simulink model "Position_augment_Testing"  (R2018a)
settings: Solver=VariableStepAuto  StartTime=0.0  StopTime=inf  RelTol=1e-3
undefined symbols (not defined in the file): Ad, Bd, Beta, C1, C2, cBW, d, dw, I, Iw, Kb, Kg, Kt, La, mc, R, Ra, sampleTime, Waypoint
libraries: cstblocks x3, mobileRoboticsLib x2, dspsrcs4 x1
settings Model: Creator=shravan  LastModifiedBy=shravan

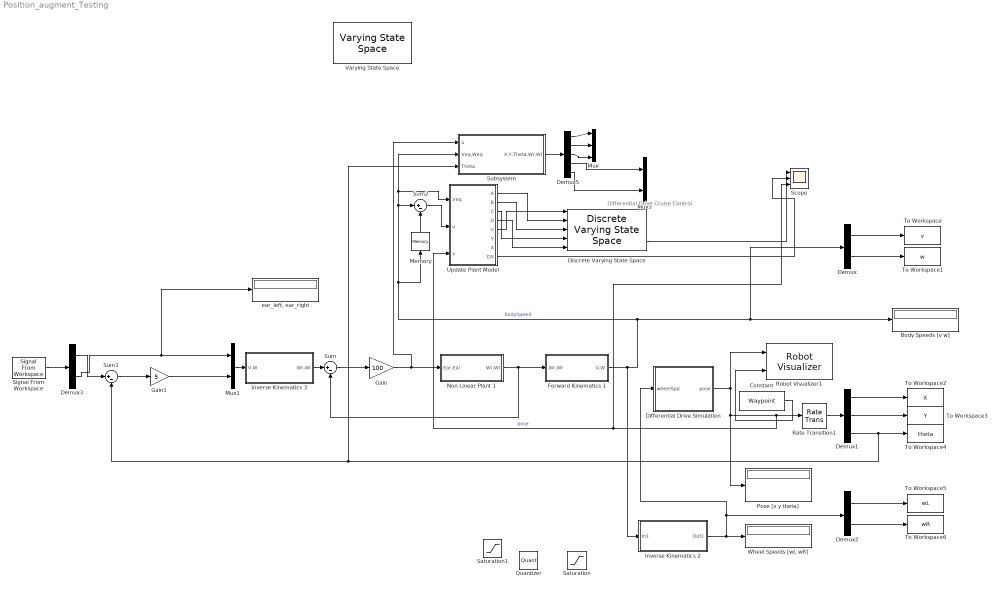
== system Position_augment_Testing ==
  note: Differential Drive Cruise Control
  Body Speeds [v w] : Display
  Constant : Constant  Value=Waypoint  SampleTime=sampleTime
  Demux : Demux  Outputs=2
  Demux1 : Demux  Outputs=3
  Demux2 : Demux  Outputs=2
  Demux3 : Demux  Outputs=2
  Demux5 : Demux  Outputs=5
  Differential Drive Simulation : Subsystem  AncestorBlock=mobileRoboticsLib/Kinematic Models/Differential Drive/Differential Drive Simulation  OverrideUsingVariant=mode==2  mask(Differential Drive Simulation){wheelRadius=R, wheelBase=dw, initX=C1, initY=C2, initAngle=0, Ts=sampleTime}
      mask prompts: wheelRadius "Wheel Radius [m]"; wheelBase "Wheelbase [m]"; initX "Initial X Position [m]"; initY "Initial Y Position [m]"; initAngle "Initial Angle [rad]"; Ts "Sample Time"
      mask help:
      | Simulates the kinematics of a differential drive vehicle from a specified initial pose.
      |
      | Input: Left and right wheel speeds [wL; wR], in rad/s
      |
      | Output: Pose [x; y; theta], in m, m, and rad
      |
      | Set the Sample Time parameter to 0 for continuous-time simulation, or a positive number for discrete-time simulation.
      mask Help: web('matlab:edit mrsDocDifferentialDrive')
      mask Callback Ts:
      | Ts = evalin('base',get_param(gcb,'Ts'));
      | blk = [gcb '/Generic Robot Simulation/Velocity Integrator'];
      | if Ts > 0
      |     set_param(blk,'OverrideUsingVariant','mode==2');
      | else
      |     set_param(blk,'OverrideUsingVariant','mode==1');
      | end
  Discrete Varying State Space : cstblocks/Linear Parameter Varying/Discrete Varying State Space  x0=[C1 C2 0]'  Ts=-1  OutputX=on  OutputDX=on
      settings: SourceProductName=Control System Toolbox  SourceProductBaseCode=CT
  Forward Kinematics 1 : Subsystem
  Gain : Gain  Gain=100
  Gain1 : Gain  Gain=5
  Inverse Kinematics 2 : Subsystem
  Inverse Kinematics 3 : Subsystem
  Memory : Memory
  Mux : Mux  Inputs=3
  Mux1 : Mux  Inputs=2
  Mux3 : Mux  Inputs=2
  Non Linear Plant 1 : Subsystem
  Pose [x y theta] : Display
  Quantizer : Quantizer
  Rate Transition1 : RateTransition  OutPortSampleTime=sampleTime
  Robot Visualizer1 : mobileRoboticsLib/Environments/Robot Visualizer  Priority=99  robotRadius=1  showTrajectory=on  hasWaypoints=on  hasLidar=off  sensorOffset=[ 0 0 ]  scanAngles=[-pi/4,0,pi/4]  hasObjDetector=off  objDetectorOffset=[ 0, 0 ]  objDetectorAngle=0  objDetectorFOV=pi/4  objDetectorMaxRange=5  objectColors=[ 1, 0, 0; 0, 1, 0; 0, 0, 1 ]  objectMarkers='s'
      settings: SourceProductName=Mobile Robotics Simulation Library
  Saturation : Saturate
  Saturation1 : Saturate  UpperLimit=12  LowerLimit=0
  Scope : Scope  NumInputPorts=3
  Signal From Workspace : dspsrcs4/Signal From Workspace  X=Cruise  Ts=cBW  nsamps=1  OutputAfterFinalValue=Holding final value  ignoreOrWarnInputAndFrameLengths=off  OutputFrames=off
  Subsystem : Subsystem
  Sum : Sum  Inputs=|+-
  Sum1 : Sum  Inputs=|+-
  Sum2 : Sum  Inputs=|+-
  To Workspace : ToWorkspace  VariableName=v  SampleTime=-1
  To Workspace1 : ToWorkspace  VariableName=w  SampleTime=-1
  To Workspace2 : ToWorkspace  VariableName=X  SampleTime=-1
  To Workspace3 : ToWorkspace  VariableName=Y  SampleTime=-1
  To Workspace4 : ToWorkspace  VariableName=theta  SampleTime=-1
  To Workspace5 : ToWorkspace  VariableName=wL  SampleTime=-1
  To Workspace6 : ToWorkspace  VariableName=wR  SampleTime=-1
  Update Plant Model : MATLAB Function  TreatAsAtomicUnit=on  SystemSampleTime=0
  Varying State Space : cstblocks/Linear Parameter Varying/Varying State Space  x0=0  xNames=''  OutputX=on  OutputDX=on
      settings: SourceProductName=Control System Toolbox
  Wheel Speeds [wL wR] : Display
  "ear_left, ear_right " : Display
  wires:
  Constant/1 -> Robot Visualizer1/2
  Differential Drive Simulation/1(pose) -> Robot Visualizer1/1, Scope/3, Update Plant Model/3(x), Rate Transition1/1, Pose [x y theta]/1  "pose"
  Sum1/1 -> Gain1/1
  Demux/1 -> To Workspace/1
  Demux/2 -> To Workspace1/1
  Demux2/1 -> To Workspace5/1
  Inverse Kinematics 3/1(Wr,Wl) -> Sum/1
  Demux1/2 -> To Workspace3/1
  Demux3/2 -> "ear_left, ear_right "/1, Mux1/1
  Rate Transition1/1 -> Demux1/1
  Forward Kinematics 1/1(V,W) -> Inverse Kinematics 2/1(In1), Memory/1, Sum2/1, Update Plant Model/1(Veq), Subsystem/2("Veq,Weq "), Demux/1, Body Speeds [v w]/1  "bodySpeed"
  Gain1/1 -> Mux1/2
  Demux2/2 -> To Workspace6/1
  Demux3/1 -> Sum1/1
  Mux1/1 -> Inverse Kinematics 3/1(V,W)
  Inverse Kinematics 2/1(Out1) -> Differential Drive Simulation/1(wheelSpd), Demux2/1, Wheel Speeds [wL wR]/1
  Demux1/1 -> To Workspace2/1
  Signal From Workspace/1 -> Demux3/1
  Subsystem/1(X,Y,Theta,Wr,Wl) -> Demux5/1
  Demux5/2 -> Mux/2
  Demux5/1 -> Mux/1
  Demux5/3 -> Mux/3
  Sum/1 -> Gain/1
  Demux5/5 -> Mux3/2
  Demux5/4 -> Mux3/1
  Gain/1 -> Subsystem/1("u "), Non Linear Plant 1/1("Ear,Eal ")
  Demux1/3 -> Subsystem/3("Theta "), Sum1/2, To Workspace4/1
  Non Linear Plant 1/1(Wr,Wl) -> Sum/2, Forward Kinematics 1/1(Wr,Wl)
  Update Plant Model/1(A) -> Discrete Varying State Space/2
  Update Plant Model/2(B) -> Discrete Varying State Space/3
  Update Plant Model/3(C) -> Discrete Varying State Space/4
  Update Plant Model/4(D) -> Discrete Varying State Space/5
  Update Plant Model/5(U) -> Discrete Varying State Space/1
  Memory/1 -> Sum2/2
  Sum2/1 -> Update Plant Model/2(u)
  Discrete Varying State Space/3 -> Scope/1
  Update Plant Model/8(DX) -> Scope/2

== system Position_augment_Testing/Differential Drive Simulation ==
  wheelSpd : Inport
  Constant : Constant  Value=0
  Demux : Demux  Outputs=2
  "Forward Kinematics " : Subsystem
  Generic Robot Simulation : mobileRoboticsLib/Utilities/Generic Vehicle Simulation  initX=initX  initY=initY  initAngle=initAngle  Ts=Ts
      link override Velocity Integrator: OverrideUsingVariant=mode==2
      settings: SourceProductName=Mobile Robotics Simulation Toolbox
  Mux1 : Mux  Inputs=3
  pose : Outport
  wires:
  Generic Robot Simulation/1 -> pose/1
  "Forward Kinematics "/1(Out1) -> Demux/1
  wheelSpd/1 -> "Forward Kinematics "/1(In1)
  Constant/1 -> Mux1/2  "vy"
  Demux/2 -> Mux1/3  "w"
  Demux/1 -> Mux1/1  "vx"
  Mux1/1 -> Generic Robot Simulation/1

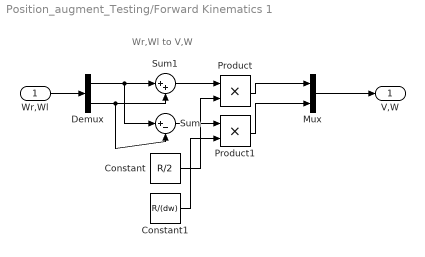
== system Position_augment_Testing/Forward Kinematics 1 ==
  note: Wr,Wl to V,W
  Wr,Wl : Inport
  Constant : Constant  Value=R/2
  Constant1 : Constant  Value=R/(dw)
  Demux : Demux  Outputs=2
  Mux : Mux  Inputs=2
  Product : Product
  Product1 : Product
  Sum : Sum  Inputs=|+-
  Sum1 : Sum  Inputs=|++
  V,W : Outport
  wires:
  Constant1/1 -> Product1/2
  Sum/1 -> Product1/1
  Constant/1 -> Product/2
  Sum1/1 -> Product/1
  Demux/2 -> Sum1/2, Sum/2
  Demux/1 -> Sum1/1, Sum/1
  Product/1 -> Mux/1
  Mux/1 -> V,W/1
  Product1/1 -> Mux/2
  Wr,Wl/1 -> Demux/1

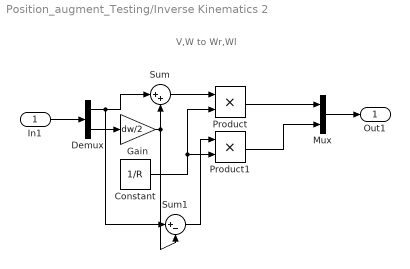
== system Position_augment_Testing/Inverse Kinematics 2 ==
  note: V,W to Wr,Wl
  In1 : Inport
  Constant : Constant  Value=1/R
  Demux : Demux  Outputs=2
  Gain : Gain  Gain=dw/2
  Mux : Mux  Inputs=2
  Product : Product
  Product1 : Product
  Sum : Sum  Inputs=|++
  Sum1 : Sum  Inputs=|+-
  Out1 : Outport
  wires:
  Gain/1 -> Sum/2, Sum1/2
  Product1/1 -> Mux/2
  Product/1 -> Mux/1
  Sum1/1 -> Product1/1
  Constant/1 -> Product/2, Product1/2
  Sum/1 -> Product/1
  Demux/1 -> Sum/1, Sum1/1
  Demux/2 -> Gain/1
  In1/1 -> Demux/1
  Mux/1 -> Out1/1

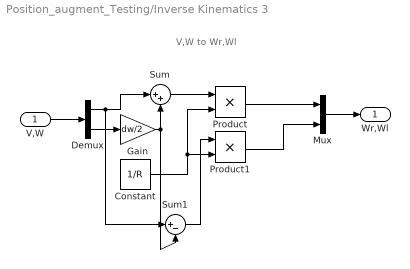
== system Position_augment_Testing/Inverse Kinematics 3 ==
  note: V,W to Wr,Wl
  V,W : Inport
  Constant : Constant  Value=1/R
  Demux : Demux  Outputs=2
  Gain : Gain  Gain=dw/2
  Mux : Mux  Inputs=2
  Product : Product
  Product1 : Product
  Sum : Sum  Inputs=|++
  Sum1 : Sum  Inputs=|+-
  Wr,Wl : Outport
  wires:
  Gain/1 -> Sum/2, Sum1/2
  Product1/1 -> Mux/2
  Product/1 -> Mux/1
  Sum1/1 -> Product1/1
  Constant/1 -> Product/2, Product1/2
  Sum/1 -> Product/1
  Demux/1 -> Sum/1, Sum1/1
  Demux/2 -> Gain/1
  V,W/1 -> Demux/1
  Mux/1 -> Wr,Wl/1

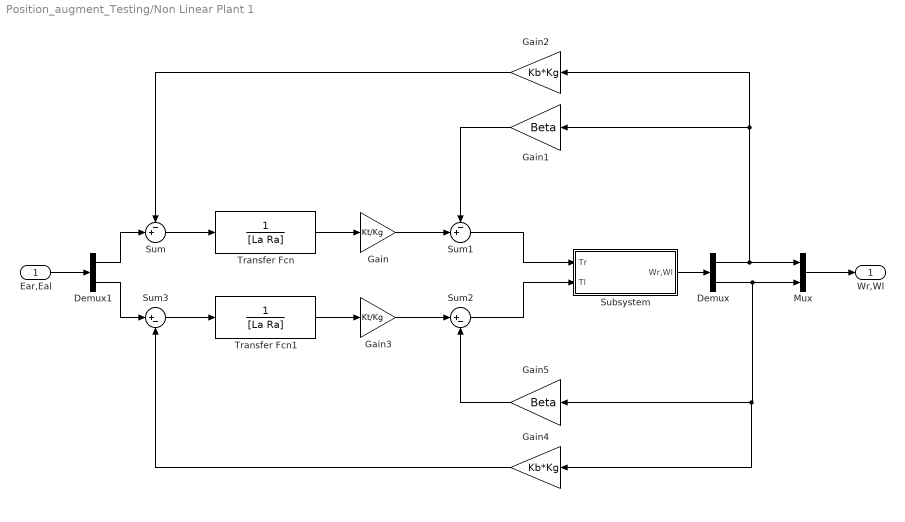
== system Position_augment_Testing/Non Linear Plant 1 ==
  "Ear,Eal " : Inport
  Demux : Demux  Outputs=2
  Demux1 : Demux  Outputs=2
  Gain : Gain  Gain=Kt/Kg
  Gain1 : Gain  Gain=Beta
  Gain2 : Gain  Gain=Kb*Kg
  Gain3 : Gain  Gain=Kt/Kg
  Gain4 : Gain  Gain=Kb*Kg
  Gain5 : Gain  Gain=Beta
  Mux : Mux  Inputs=2
  Subsystem : Subsystem
  Sum : Sum  Inputs=-+|
  Sum1 : Sum  Inputs=-+|
  Sum2 : Sum  Inputs=|+-
  Sum3 : Sum  Inputs=|+-
  Transfer Fcn : TransferFcn  Denominator=[La Ra]
  Transfer Fcn1 : TransferFcn  Denominator=[La Ra]
  Wr,Wl : Outport
  wires:
  Sum2/1 -> Subsystem/2(Tl)
  Demux/2 -> Gain5/1, Gain4/1, Mux/2
  Gain3/1 -> Sum2/1
  Transfer Fcn1/1 -> Gain3/1
  Transfer Fcn/1 -> Gain/1
  Sum1/1 -> Subsystem/1(Tr)
  "Ear,Eal "/1 -> Demux1/1
  Gain/1 -> Sum1/2
  Gain2/1 -> Sum/1
  Mux/1 -> Wr,Wl/1
  Sum3/1 -> Transfer Fcn1/1
  Demux1/1 -> Sum/2
  Subsystem/1(Wr,Wl) -> Demux/1
  Demux/1 -> Gain1/1, Gain2/1, Mux/1
  Gain1/1 -> Sum1/1
  Demux1/2 -> Sum3/1
  Sum/1 -> Transfer Fcn/1
  Gain4/1 -> Sum3/2
  Gain5/1 -> Sum2/2

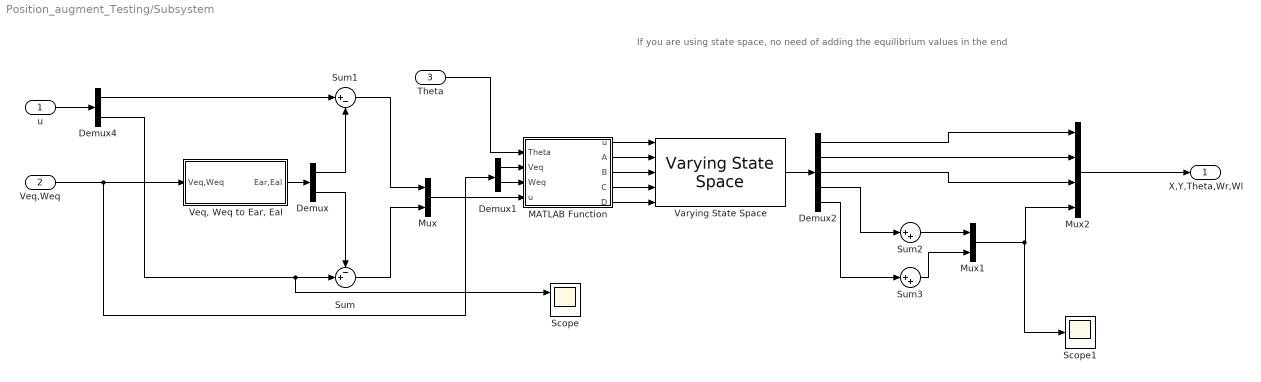
== system Position_augment_Testing/Subsystem ==
  note: If you are using state space, no need of adding the equilibrium values in the end
  "u " : Inport
  "Veq,Weq " : Inport  Port=2
  "Theta " : Inport  Port=3
  Demux : Demux  Outputs=2
  Demux1 : Demux  Outputs=2
  Demux2 : Demux  Outputs=5
  Demux4 : Demux  Outputs=2
  MATLAB Function : MATLAB Function  TreatAsAtomicUnit=on  SystemSampleTime=sampleTime*0.1
  Mux : Mux  Inputs=2
  Mux1 : Mux  Inputs=2
  Mux2 : Mux
  Scope : Scope  NumInputPorts=2
  Scope1 : Scope
  Sum : Sum  Inputs=-+|
  Sum1 : Sum  Inputs=|+-
  Sum2 : Sum  Inputs=|++
  Sum3 : Sum  Inputs=|++
  Varying State Space : cstblocks/Linear Parameter Varying/Varying State Space  x0=[C1;C2;0;0;0;0;0]  xNames=''  OutputX=off  OutputDX=off
      settings: SourceProductName=Control System Toolbox
  "Veq, Weq to Ear, Eal " : Subsystem
  X,Y,Theta,Wr,Wl : Outport
  wires:
  "Veq, Weq to Ear, Eal "/1(Ear,Eal) -> Demux/1
  Demux/1 -> Sum1/2
  Demux/2 -> Sum/1
  MATLAB Function/3(B) -> Varying State Space/3
  MATLAB Function/4(C) -> Varying State Space/4
  MATLAB Function/1(u) -> Varying State Space/1
  MATLAB Function/2(A) -> Varying State Space/2
  MATLAB Function/5(D) -> Varying State Space/5
  Sum1/1 -> Mux/1
  Sum/1 -> Mux/2
  Mux/1 -> MATLAB Function/4("u ")
  "Theta "/1 -> MATLAB Function/1(Theta)
  Demux1/2 -> MATLAB Function/3(Weq)
  Demux1/1 -> MATLAB Function/2(Veq)
  Varying State Space/1 -> Demux2/1
  Demux2/1 -> Mux2/1
  Demux2/2 -> Mux2/2
  Demux2/3 -> Mux2/3
  Demux2/4 -> Sum2/1
  Demux2/5 -> Sum3/1
  Mux1/1 -> Scope1/1, Mux2/4
  Sum2/1 -> Mux1/1
  Sum3/1 -> Mux1/2
  "Veq,Weq "/1 -> "Veq, Weq to Ear, Eal "/1(Veq,Weq), Demux1/1
  Mux2/1 -> X,Y,Theta,Wr,Wl/1
  "u "/1 -> Demux4/1
  Demux4/1 -> Sum1/1
  Demux4/2 -> Scope/1, Sum/2

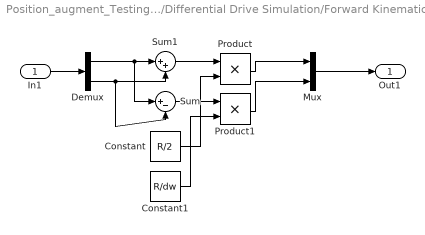
== system Position_augment_Testing/Differential Drive Simulation/Forward Kinematics  ==
  In1 : Inport
  Constant : Constant  Value=R/2
  Constant1 : Constant  Value=R/dw
  Demux : Demux  Outputs=2
  Mux : Mux  Inputs=2
  Product : Product
  Product1 : Product
  Sum : Sum  Inputs=|+-
  Sum1 : Sum  Inputs=|++
  Out1 : Outport
  wires:
  In1/1 -> Demux/1
  Product1/1 -> Mux/2
  Mux/1 -> Out1/1
  Product/1 -> Mux/1
  Demux/1 -> Sum/1, Sum1/1
  Demux/2 -> Sum/2, Sum1/2
  Sum1/1 -> Product/1
  Constant/1 -> Product/2
  Sum/1 -> Product1/1
  Constant1/1 -> Product1/2

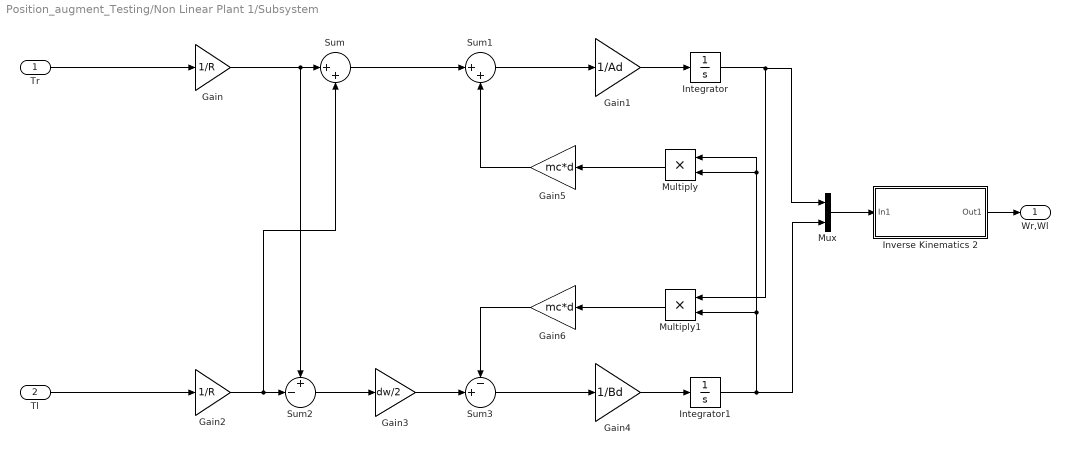
== system Position_augment_Testing/Non Linear Plant 1/Subsystem ==
  Tr : Inport
  Tl : Inport  Port=2
  Gain : Gain  Gain=1/R
  Gain1 : Gain  Gain=1/Ad
  Gain2 : Gain  Gain=1/R
  Gain3 : Gain  Gain=dw/2
  Gain4 : Gain  Gain=1/Bd
  Gain5 : Gain  Gain=mc*d
  Gain6 : Gain  Gain=mc*d
  Integrator : Integrator
  Integrator1 : Integrator
  Inverse Kinematics 2 : Subsystem
  Multiply : Product
  Multiply1 : Product
  Mux : Mux  Inputs=2
  Sum : Sum  Inputs=|++
  Sum1 : Sum  Inputs=|++
  Sum2 : Sum  Inputs=+-|
  Sum3 : Sum  Inputs=-+|
  Wr,Wl : Outport
  wires:
  Gain1/1 -> Integrator/1
  Tl/1 -> Gain2/1
  Gain6/1 -> Sum3/1
  Gain2/1 -> Sum2/2, Sum/2
  Sum2/1 -> Gain3/1
  Gain3/1 -> Sum3/2
  Multiply/1 -> Gain5/1
  Integrator1/1 -> Mux/2, Multiply/1, Multiply/2, Multiply1/2
  Tr/1 -> Gain/1
  Gain5/1 -> Sum1/2
  Sum/1 -> Sum1/1
  Inverse Kinematics 2/1(Out1) -> Wr,Wl/1
  Gain4/1 -> Integrator1/1
  Mux/1 -> Inverse Kinematics 2/1(In1)
  Integrator/1 -> Multiply1/1, Mux/1
  Gain/1 -> Sum2/1, Sum/1
  Sum3/1 -> Gain4/1
  Multiply1/1 -> Gain6/1
  Sum1/1 -> Gain1/1

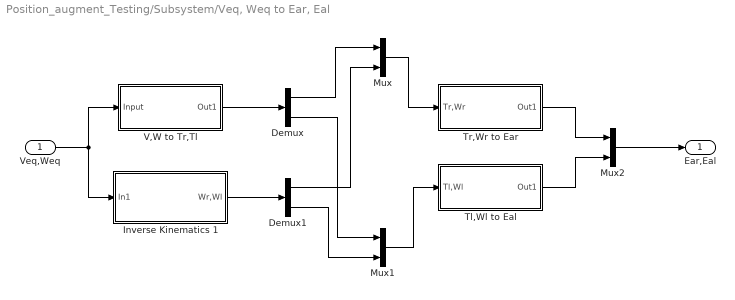
== system Position_augment_Testing/Subsystem/Veq, Weq to Ear, Eal  ==
  Veq,Weq : Inport
  Demux : Demux  Outputs=2
  Demux1 : Demux  Outputs=2
  Inverse Kinematics 1 : Subsystem
  Mux : Mux  Inputs=2
  Mux1 : Mux  Inputs=2
  Mux2 : Mux  Inputs=2
  Tl,Wl to Eal : Subsystem
  Tr,Wr to Ear : Subsystem
  V,W to Tr,Tl : Subsystem
  Ear,Eal : Outport
  wires:
  V,W to Tr,Tl/1(Out1) -> Demux/1
  Demux/1 -> Mux/1
  Mux/1 -> Tr,Wr to Ear/1(Tr,Wr)
  Veq,Weq/1 -> Inverse Kinematics 1/1(In1), V,W to Tr,Tl/1(Input)
  Inverse Kinematics 1/1(Wr,Wl) -> Demux1/1
  Demux1/1 -> Mux/2
  Demux/2 -> Mux1/1
  Demux1/2 -> Mux1/2
  Mux1/1 -> Tl,Wl to Eal/1(Tl,Wl)
  Tr,Wr to Ear/1(Out1) -> Mux2/1
  Tl,Wl to Eal/1(Out1) -> Mux2/2
  Mux2/1 -> Ear,Eal/1

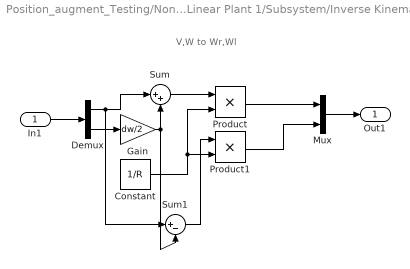
== system Position_augment_Testing/Non Linear Plant 1/Subsystem/Inverse Kinematics 2 ==
  note: V,W to Wr,Wl
  In1 : Inport
  Constant : Constant  Value=1/R
  Demux : Demux  Outputs=2
  Gain : Gain  Gain=dw/2
  Mux : Mux  Inputs=2
  Product : Product
  Product1 : Product
  Sum : Sum  Inputs=|++
  Sum1 : Sum  Inputs=|+-
  Out1 : Outport
  wires:
  Product1/1 -> Mux/2
  Product/1 -> Mux/1
  Sum1/1 -> Product1/1
  Constant/1 -> Product/2, Product1/2
  Sum/1 -> Product/1
  Gain/1 -> Sum/2, Sum1/2
  Demux/1 -> Sum/1, Sum1/1
  Demux/2 -> Gain/1
  In1/1 -> Demux/1
  Mux/1 -> Out1/1

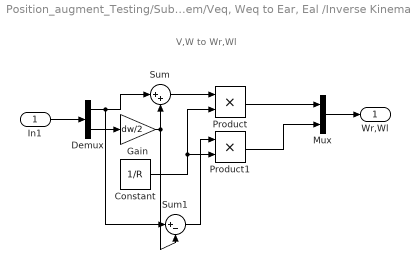
== system Position_augment_Testing/Subsystem/Veq, Weq to Ear, Eal /Inverse Kinematics 1 ==
  note: V,W to Wr,Wl
  In1 : Inport
  Constant : Constant  Value=1/R
  Demux : Demux  Outputs=2
  Gain : Gain  Gain=dw/2
  Mux : Mux  Inputs=2
  Product : Product
  Product1 : Product
  Sum : Sum  Inputs=|++
  Sum1 : Sum  Inputs=|+-
  Wr,Wl : Outport
  wires:
  Mux/1 -> Wr,Wl/1
  In1/1 -> Demux/1
  Demux/2 -> Gain/1
  Demux/1 -> Sum1/1, Sum/1
  Sum/1 -> Product/1
  Constant/1 -> Product1/2, Product/2
  Sum1/1 -> Product1/1
  Product/1 -> Mux/1
  Product1/1 -> Mux/2
  Gain/1 -> Sum1/2, Sum/2

== system Position_augment_Testing/Subsystem/Veq, Weq to Ear, Eal /Tl,Wl to Eal ==
  Tl,Wl : Inport
  Demux1 : Demux  Outputs=2
  Gain : Gain  Gain=Ra*Kg/Kt
  Gain1 : Gain  Gain=Beta
  Gain2 : Gain  Gain=Ra*Kg/Kt
  Gain3 : Gain  Gain=Kb*Kg
  Sum : Sum  Inputs=|+++
  Out1 : Outport
  wires:
  Gain1/1 -> Sum/2
  Gain2/1 -> Gain1/1
  Gain/1 -> Sum/1
  Gain3/1 -> Sum/3
  Sum/1 -> Out1/1
  Tl,Wl/1 -> Demux1/1
  Demux1/1 -> Gain/1
  Demux1/2 -> Gain3/1, Gain2/1

== system Position_augment_Testing/Subsystem/Veq, Weq to Ear, Eal /Tr,Wr to Ear ==
  Tr,Wr : Inport
  Demux1 : Demux  Outputs=2
  Gain : Gain  Gain=Ra*Kg/Kt
  Gain1 : Gain  Gain=Beta
  Gain2 : Gain  Gain=Ra*Kg/Kt
  Gain3 : Gain  Gain=Kb*Kg
  Sum : Sum  Inputs=|+++
  Out1 : Outport
  wires:
  Gain2/1 -> Gain1/1
  Tr,Wr/1 -> Demux1/1
  Sum/1 -> Out1/1
  Gain1/1 -> Sum/2
  Gain3/1 -> Sum/3
  Demux1/2 -> Gain3/1, Gain2/1
  Gain/1 -> Sum/1
  Demux1/1 -> Gain/1

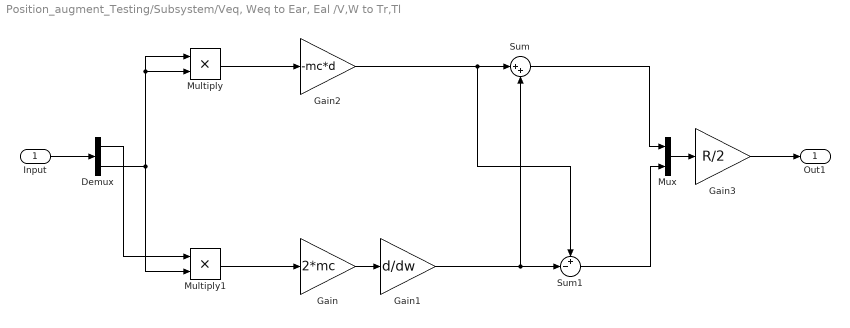
== system Position_augment_Testing/Subsystem/Veq, Weq to Ear, Eal /V,W to Tr,Tl ==
  Input : Inport
  Demux : Demux  Outputs=2
  Gain : Gain  Gain=2*mc
  Gain1 : Gain  Gain=d/dw
  Gain2 : Gain  Gain=-mc*d
  Gain3 : Gain  Gain=R/2
  Multiply : Product
  Multiply1 : Product
  Mux : Mux  Inputs=2
  Sum : Sum  Inputs=|++
  Sum1 : Sum  Inputs=+-|
  Out1 : Outport
  wires:
  Demux/1 -> Multiply1/1
  Mux/1 -> Gain3/1
  Gain/1 -> Gain1/1
  Input/1 -> Demux/1
  Multiply1/1 -> Gain/1
  Sum1/1 -> Mux/2
  Gain1/1 -> Sum1/2, Sum/2
  Gain2/1 -> Sum1/1, Sum/1
  Demux/2 -> Multiply1/2, Multiply/2, Multiply/1
  Gain3/1 -> Out1/1
  Multiply/1 -> Gain2/1
  Sum/1 -> Mux/1

== matlab function Position_augment_Testing/Update Plant Model ==
  data: Veq input; u input size=[2,1]; A output size=[3,3]; x input size=[3,1]; B output size=[3,2]; C output size=[3,3]; D output size=[3,2]; U output size=[2,1]; Y output size=[3,1]; X output size=[3,1]; DX output size=[3,1]
function [A,B,C,D,U,Y,X,DX] = fcn(Veq,u,x)
% Sample time
Ts = 0.01;

% Model parameters
U1eq = Veq(1);
Thetaeq = x(3);

% Continuous-time model
Ac = [0 0 -U1eq*sin(Thetaeq);
      0 0  U1eq*cos(Thetaeq);
      0 0  0];
Bc = [cos(Thetaeq) 0;
      sin(Thetaeq) 0;
      0            1];   
Cc = [1 0 0; 0 1 0; 0 0 1];
Dc = zeros(3,2);

% Generate discrete-time model
nx = size(Ac,1);
nu = size(Bc,2);
M = expm([[Ac Bc]*Ts; zeros(nu,nx+nu)]);
A = Ac%M(1:nx,1:nx);
B = Bc%M(1:nx,nx+1:nx+nu);
C = Cc;
D = Dc;

% Nominal conditions for discrete-time plant
X = x;
U = u;
Y = C*x + D*u;
DX = A*x+B*u-x;

== matlab function Position_augment_Testing/Subsystem/MATLAB Function ==
  data: Theta input size=[1,1]; Veq input size=[1,1]; Weq input size=[1,1]; u input size=[2,1]; u output; A output; B output; C output; D output; sampleTime parameter; I parameter; Iw parameter; R parameter
function [u,A,B,C,D] = fcn(Theta,Veq,Weq,u,sampleTime,I, Iw,R)
% Sample time
Ts = sampleTime;
d = 0.0107; L = 0.28; AR = L/0.25; dw = 0.25; md = 0;
d = 0; thetaeq = Theta;
% Model Parameters
Kt = 0.0046; Kg = 50; Kb = Kt; Beta = 2.29e-06; La =1.729e-03; Ra = 5.51;
m = 3.4; mc = 2.76 + md; I = I ; Iw = Iw; L = L; d = d; dw = dw; 
Ao = m + 2*Iw/(R*R); Bo = I + dw*dw*Iw/(2*R*R);

% Continuous-time model for Plant e_r, e_l to Wr,Wl
% ULTIMATE - CORRECT representation of Plant using State Space form derived
% on Aug 24 th, 2020 
Ac = [-2*Beta/(Ao*R*R) 2*mc*d*Weq/Ao   (Kt/(Kg*R*Ao))  (Kt/(Kg*R*Ao));
     -mc*d*Weq/Bo  (-mc*d*Veq/Bo)-(Beta*dw*dw/(2*R*R*Bo)) dw*Kt/(2*Kg*R*Bo) -dw*Kt/(2*Kg*Bo*R) ;
     -Kb*Kg/(La*R)   -Kb*Kg*dw/(2*La*R)  -Ra/La      0 ;
     -Kb*Kg/(La*R)    Kb*Kg*dw/(2*La*R)    0       -Ra/La ];
Bc = [0 0; 0 0; 1/La 0; 0 1/La]; Cc =  [1/R dw/(2*R); 1/R -dw/(2*R)]*[1 0 0 0; 0 1 0 0]; Dc = [0 0;0 0];


% States x,y,theta, V,W, Iar,Ial 

Au =      [0  0  -Veq*sin(thetaeq) cos(thetaeq)  0  0  0;
           0  0  Veq*cos(thetaeq) sin(thetaeq)  0  0  0;
           0  0  0                 0            1  0  0;  
           zeros(4,3) Ac]
Bu =      [0 0;
           0 0;
           0 0;
           Bc]
Cu =      [1 0 0 0 0 0 0;
           0 1 0 0 0 0 0;
           0 0 1 0 0 0 0;
           zeros(2,3) Cc]
Du =       zeros(5,2)

% Discretize the continuous-time model using zero-order hold 
% on the inputs and a sample time of Ts seconds
nx = size(Au,1);
nu = size(Bu,2);
M = expm([[Au Bu]*Ts; zeros(nu,nx+nu)]);
A = Au;%M(1:nx,1:nx);
B = Bu;%M(1:nx,nx+1:nx+nu);
C = Cu;
D = Du;

% Nominal conditions for discrete-time plant
%X = x;
u = u;
%Y = Co*x + Do*u;
%DX = Ao*x+Bo*u-x;
%y = u;
